simulink model "slopeofequation"  (R2020b)
settings: Solver=VariableStepAuto  StartTime=0.0  StopTime=10.0  RelTol=1e-3
settings Model: Creator=99003736  LastModifiedBy=99003736

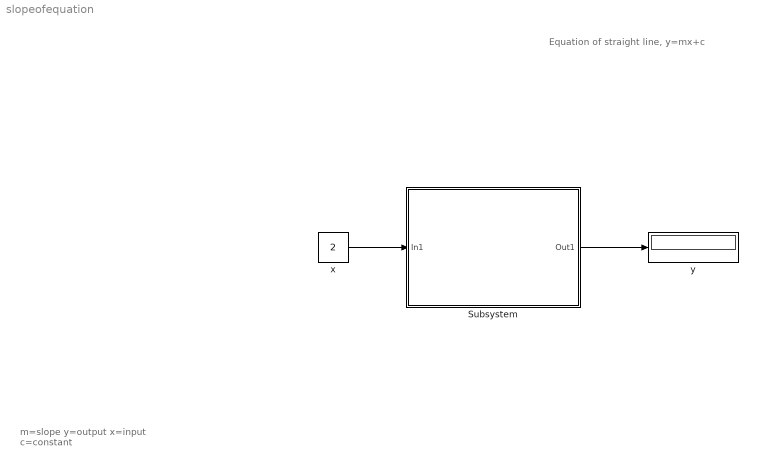
== system slopeofequation ==
  note: m=slope
      | y=output
      | x=input
      | c=constant
  note: Equation of straight line, y=mx+c
  Subsystem : Subsystem  mask(subsystem straight line){m=5, c=2}
      mask prompts: m "slope of line"; c "constant"
      mask help: this is a susbsystem for equation of straight line
      mask Help: www.ltts.com
      mask Display: image('C:\Users\99003736\Desktop\the-equation-of-a-straight-line-l.jpg')
  x : Constant  Value=2
  y : Display
  wires:
  x/1 -> Subsystem/1(In1)
  Subsystem/1(Out1) -> y/1

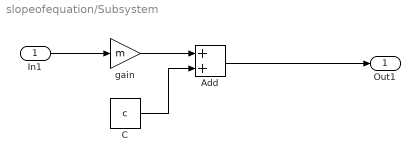
== system slopeofequation/Subsystem ==
  In1 : Inport
  Add : Sum
  C : Constant  Value=c
  gain : Gain  Gain=m
  Out1 : Outport
  wires:
  In1/1 -> gain/1
  Add/1 -> Out1/1
  C/1 -> Add/2
  gain/1 -> Add/1
